simulink model "template_CR1_PreRTHS"  (Simulink 8.2)
settings: Solver=FixedStepDiscrete  StartTime=0.0  StopTime=RunningTime  FixedStep=sample  RelTol=1e-3
undefined symbols (not defined in the file): ElementsStruct, Integrator, NumFreeDOF, RigidLinkMasterMatrix, RigidLinkNo, RigidLinkNodeID, RigidLinkSlaveMatrix, sample, SampleRate, Structure
libraries: HybridFEMLibrary x2
(part 2 of 2)

== matlab function Numerical Element Calculations ==
  data: Total_RF output double; NumFreeDOF parameter double; Displacement input double; Velocity input double; ElementsStruct parameter Bus: ElementStructBus; RigidLinkNo parameter double; RigidLinkNodeID parameter double; RigidLinkMasterMatrix parameter double; RigidLinkSlaveMatrix parameter double; ElementRFs output Bus: ElementRecorderBus
% Get restoring force for each element
% Returns (6x1) restoring force vector of all elements in global coordinates %*fs
function [Total_RF,ElementRFs] = eml(NumFreeDOF, Displacement, Velocity, ElementsStruct, RigidLinkNo, RigidLinkNodeID, RigidLinkMasterMatrix, RigidLinkSlaveMatrix) %*fe
    % Store the Elements in memory
    persistent Elements;
    persistent TotalRF;        
    if isempty(Elements)
        Elements = ElementsStruct;        
    end
    
    % Storage for the Global Restoring Force        
    TotalRF = zeros(NumFreeDOF, 1);     
    ElementRFs = struct;   
    ElementRFs.Recorders = 0;
    
%Elements  %*s
[Elements.Element1, ElementRF] = GetRestoringForce_Type6(Elements.Element1, Displacement, RigidLinkNo, RigidLinkNodeID, RigidLinkMasterMatrix, RigidLinkSlaveMatrix);
TotalRF = AssembleElementGlobalRF6DOF(Elements.Element1, ElementRF, TotalRF);
[Elements.Element2, ElementRF] = GetRestoringForce_Type6(Elements.Element2, Displacement, RigidLinkNo, RigidLinkNodeID, RigidLinkMasterMatrix, RigidLinkSlaveMatrix);
TotalRF = AssembleElementGlobalRF6DOF(Elements.Element2, ElementRF, TotalRF);
[Elements.Element3, ElementRF] = GetRestoringForce_Type6(Elements.Element3, Displacement, RigidLinkNo, RigidLinkNodeID, RigidLinkMasterMatrix, RigidLinkSlaveMatrix);
TotalRF = AssembleElementGlobalRF6DOF(Elements.Element3, ElementRF, TotalRF);
[Elements.Element4, ElementRF] = GetRestoringForce_Type6(Elements.Element4, Displacement, RigidLinkNo, RigidLinkNodeID, RigidLinkMasterMatrix, RigidLinkSlaveMatrix);
TotalRF = AssembleElementGlobalRF6DOF(Elements.Element4, ElementRF, TotalRF);
[Elements.Element5, ElementRF] = GetRestoringForce_Type4(Elements.Element5, Displacement, RigidLinkNo, RigidLinkNodeID, RigidLinkMasterMatrix, RigidLinkSlaveMatrix);
TotalRF = AssembleElementGlobalRF6DOF(Elements.Element5, ElementRF, TotalRF);

%*e
                         
    Total_RF = TotalRF;


end


%%%%%%%%%%%%%%%%%%%%%%%%%%%%%%%%%%%%%%%%%%%%%%%%%%%%%%%%%%%%%%%%%%%%%%%%%%%
function TotalRF = AssembleElementGlobalRF6DOF(Element, ElementRF, TotalRF)
    % Assemble the structure restoring force vector based on the
    % degrees of freedom node locations.  
    ndof = 6;
    dof6 = zeros(6,1); 
    dof6(1,1)=Element.Nodes(1).UX;
    dof6(2,1)=Element.Nodes(1).UY;
    dof6(3,1)=Element.Nodes(1).THETA;
    dof6(4,1)=Element.Nodes(2).UX;
    dof6(5,1)=Element.Nodes(2).UY;
    dof6(6,1)=Element.Nodes(2).THETA;      

    % Add to the TotalRF    
    i = 1;
    for i=1:ndof
        if dof6(i,1) ~= -1
          TotalRF(dof6(i,1), 1) = ElementRF(i, 1) + TotalRF(dof6(i,1), 1);
        end
    end    
end

function TotalRF = AssembleElementGlobalRF9DOF(Element, ElementRF, TotalRF)
    % Assemble the structure restoring force vector based on the
    % degrees of freedom node locations.  
    ndof = 12;
    dof12 = zeros(12,1); 
    dof12(1,1)=Element.Nodes(1).UX;
    dof12(2,1)=Element.Nodes(1).UY;
    dof12(3,1)=Element.Nodes(1).THETA;
    dof12(4,1)=Element.Nodes(2).UX;
    dof12(5,1)=Element.Nodes(2).UY;
    dof12(6,1)=Element.Nodes(2).THETA;  
    dof12(7,1)=Element.Nodes(3).UX;
    dof12(8,1)=Element.Nodes(3).UY;
    dof12(9,1)=Element.Nodes(3).THETA;
    dof12(10,1)=Element.Nodes(4).UX;
    dof12(11,1)=Element.Nodes(4).UY;
    dof12(12,1)=Element.Nodes(4).THETA;

    % Add to the TotalRF
    for i=1:ndof
        if dof12(i,1) ~= -1
          TotalRF(dof12(i,1), 1) = ElementRF(i, 1) + TotalRF(dof12(i,1), 1);
        end
    end    
end

%% Element 1
function [Element, RestoringForce] = GetRestoringForce_Type1(Element, Displacement, RigidLinkNo, RigidLinkNodeID, RigidLinkMasterMatrix, RigidLinkSlaveMatrix)
    % Get distance between nodes
    X21 = Element.Nodes(2).Xcoord - Element.Nodes(1).Xcoord;
    Y21 = Element.Nodes(2).Ycoord - Element.Nodes(1).Ycoord;
    EL = sqrt(X21 * X21 + Y21 * Y21);
    EAL = Element.Material.E * Element.Area / EL;
    EIZL = Element.Material.E * Element.Inertia / EL;    
    % Calculation of density (the uniform load is only taken into account)
    SEP = zeros(6);
    SEP(1, 1) = EAL;
    SEP(1, 4) = -EAL;
    SEP(4, 4) = EAL;
    SEP(2, 2) = 12 * EIZL / EL ^ 2;
    SEP(2, 3) = 6 * EIZL / EL;
    SEP(2, 5) = -SEP(2, 2);
    SEP(2, 6) = SEP(2, 3);
    SEP(3, 3) = 4 * EIZL;
    SEP(3, 5) = -6 * EIZL / EL;
    SEP(3, 6) = 2 * EIZL;
    SEP(5, 5) = 12 * EIZL / EL ^ 2;
    SEP(5, 6) = -6 * EIZL / EL;
    SEP(6, 6) = 4 * EIZL;
    for i = 1:6
       for j = i:6
          SEP(j, i) = SEP(i, j);
       end
    end
    DCOS = zeros(3);
    DCOS(1, 1) = X21 / EL;
    DCOS(1, 2) = Y21 / EL;
    DCOS(1, 3) = 0;
    DCOS(2, 1) = -DCOS(1, 2);
    DCOS(2, 2) = DCOS(1, 1);
    DCOS(2, 3) = 0;
    DCOS(3, 1) = 0;
    DCOS(3, 2) = 0;
    DCOS(3, 3) = 1;
    ALMBDA = zeros(6);       
    for i = 1:2
       IK = 3 * (i - 1);
       for j = 1:3
          for k = 1:3
             ALMBDA(j + IK, k + IK) = DCOS(j, k);
          end
       end
    end
    SE = ALMBDA' * SEP * ALMBDA;
    % Create the displacement Ue (6x1) vector of the element in global coordinates
    Ue = zeros(6,1);
    dof = zeros(6,1);
    dof(1,1)=Element.Nodes(1).UX;
    dof(2,1)=Element.Nodes(1).UY;
    dof(3,1)=Element.Nodes(1).THETA;
    dof(4,1)=Element.Nodes(2).UX;
    dof(5,1)=Element.Nodes(2).UY;
    dof(6,1)=Element.Nodes(2).THETA;
    
    for i=1:6
        if dof(i,1) ~= -1
            Ue(i,1)=Displacement(dof(i,1),1);
        end
    end

    % Calculation Restoring Force, considering the Rigid Links if used
    if( RigidLinkNo )
        TR = RigidLinkTransformation2Nodes(Element.Nodes(1).ID, Element.Nodes(2).ID, RigidLinkNo, RigidLinkNodeID, RigidLinkMasterMatrix, RigidLinkSlaveMatrix);
        RestoringForce = TR' * SE * TR * Ue;  % (6x1) resisting force vector of element in global coordinates
    else        
        RestoringForce = SE * Ue;  % (6x1) resisting force vector of element in global coordinates
    end
end

%% Element 2
function [Element, RestoringForce] = GetRestoringForce_Type2(Element, Displacement, RigidLinkNo, RigidLinkNodeID, RigidLinkMasterMatrix, RigidLinkSlaveMatrix)
    % Preset arrays
    SE = zeros(6,6);
    SE(1, 1) = Element.Stiffness;
    SE(1, 4) = -Element.Stiffness;
    SE(4, 4) = Element.Stiffness;
    SE(4, 1) = SE(1,4);
    
    % Create the displacement Ue (6x1) vector of the element in global coordinates
    Ue = zeros(6,1);
    dof = zeros(6,1);
    dof(1,1)=Element.Nodes(1).UX;
    dof(2,1)=Element.Nodes(1).UY;
    dof(3,1)=Element.Nodes(1).THETA;
    dof(4,1)=Element.Nodes(2).UX;
    dof(5,1)=Element.Nodes(2).UY;
    dof(6,1)=Element.Nodes(2).THETA;
    
    for i=1:6
        if dof(i,1) ~= -1
            Ue(i,1)=Displacement(dof(i,1),1);
        end
    end

    % Calculation Restoring Force, considering the Rigid Links if used
    if( RigidLinkNo )
        TR = RigidLinkTransformation2Nodes(Element.Nodes(1).ID, Element.Nodes(2).ID, RigidLinkNo, RigidLinkNodeID, RigidLinkMasterMatrix, RigidLinkSlaveMatrix);
        RestoringForce = TR' * SE * TR * Ue;  % (6x1) resisting force vector of element in global coordinates
    else
%         if (RUNMODE_BIT)
%             RestoringForce = zeros(6,1);
%             RestoringForce(1,1) = Element2Input;
%             RestoringForce(4,1) = -Element2Input;
%         else
            RestoringForce = SE * Ue;  % (6x1) resisting force vector of element in global coordinates
%         end
    end    
end

%% Element 3

%% Element 4
function [Element, RestoringForce] = GetRestoringForce_Type4(Element, Displacement, RigidLinkNo, RigidLinkNodeID, RigidLinkMasterMatrix, RigidLinkSlaveMatrix)

    % element geometry       
    % element deformation % geometry restricted to 1,2 plane (x,y)
    dx = Element.xyj(1,1) - Element.xyi(1,1); 
    dy = Element.xyj(2,1) - Element.xyi(2,1);
    L = sqrt(dx*dx+dy*dy);
    dx = dx / L;
    dy = dy / L;

    % 6x6 transformation matrix from local to global coordiante
    apq  = zeros(6);
    apq(1,1) = dx; apq(2,2) = dx; apq(4,4) = dx; apq(5,5)= dx;
    apq(1,2) = dy; apq(2,1) =-dy; apq(4,5) = dy; apq(5,4)=-dy;
    apq(3,3) = 1.0; apq(6,6) =1.0;

    % element stiffness matrix in local coordinate
    SE = zeros(6,6);  
    SE(2, 2) = Element.K22;
    SE(2, 5) = Element.K25;
    SE(5, 2) = Element.K52;
    SE(5, 5) = Element.K55;
    % transformed element stiffness matrix in global coordinate
    SE = apq' * SE * apq;

    % Create the displacement Ue (6x1) vector of the element in global coordinates
    Ue = zeros(6,1);
    dof = zeros(6,1);
    dof(1,1)=Element.Nodes(1).UX;
    dof(2,1)=Element.Nodes(1).UY;
    dof(3,1)=Element.Nodes(1).THETA;
    dof(4,1)=Element.Nodes(2).UX;
    dof(5,1)=Element.Nodes(2).UY;
    dof(6,1)=Element.Nodes(2).THETA;

    for i=1:6
        if dof(i,1) ~= -1
            Ue(i,1) = Displacement(dof(i,1),1);
        end
    end
    
    % Calculation Restoring Force, considering the Rigid Links if used
    if( RigidLinkNo )
        TR = RigidLinkTransformation2Nodes(Element.Nodes(1).ID, Element.Nodes(2).ID, RigidLinkNo, RigidLinkNodeID, RigidLinkMasterMatrix, RigidLinkSlaveMatrix);
        RestoringForce = TR' * SE * TR * Ue;  % (6x1) resisting force vector of element in global coordinates
    else
        RestoringForce = SE * Ue;  % (6x1) resisting force vector of element in global coordinates
    end
end

%% Element 5

%% Element 6
function [Element,RestoringForce] = GetRestoringForce_Type6(Element, Displacement, RigidLinkNo, RigidLinkNodeID, RigidLinkMasterMatrix, RigidLinkSlaveMatrix)
    % Get the displacement Ue (6x1) vector of the element in global coordinates
    Ue = zeros(6,1);
    dof=zeros(6,1);
    dof(1,1)=Element.Nodes(1).UX;
    dof(2,1)=Element.Nodes(1).UY;
    dof(3,1)=Element.Nodes(1).THETA;
    dof(4,1)=Element.Nodes(2).UX;
    dof(5,1)=Element.Nodes(2).UY;
    dof(6,1)=Element.Nodes(2).THETA;
    for i=1:6
        if dof(i,1) ~= -1
            Ue(i,1)=Displacement(dof(i,1),1);
        end
    end

    % Calculation Restoring Force, considering the Rigid Links if used
    if( RigidLinkNo )
        TR = RigidLinkTransformation2Nodes(Element.Nodes(1).ID, Element.Nodes(2).ID, RigidLinkNo, RigidLinkNodeID, RigidLinkMasterMatrix, RigidLinkSlaveMatrix);        
        Ue = TR * Ue; 
    end       

    du=Ue-Element.Uprev;  % The incremental displacement vector du of the element in global coordinates 
    Element.Uprev=Ue; %Update Uprev of element for use in next state determination call

    % Incremental basic deformations
    dv = Element.avq * du;      

    % Integrate basic force and basic stiffness matrix
    kb = zeros(3);
    s  = zeros(3,1);

    for i=1:length(Element.sections)

        % Form B matrix and compute section deformation
        B = [ Element.b1(i) Element.b2(i) 0; 0 0 Element.b3(i) ];
        dvs = B * dv;  

        % Section state determination and update section state
        [ss ks Element.sections(i)] = SectionState( Element.sections(i), dvs );

        % Sum section term
        kb = kb + B'*ks*B * ( Element.wi(i) * Element.L/2 );
        s  = s  + B'*ss   * ( Element.wi(i) * Element.L/2 );

    end

    % Restoring force and stiffness matrix
    RestoringForce = Element.avq' * s;

    if( RigidLinkNo )
        RestoringForce = TR' * RestoringForce;  
    end
end

%% Element 7
function [Element,RestoringForce] = GetRestoringForce_Type7(Element, Displacement, RigidLinkNo, RigidLinkNodeID, RigidLinkMasterMatrix, RigidLinkSlaveMatrix, maxIter, EAT, ERT, CO)
    % Get the displacement Ue (6x1) vector of the element in global coordinates
    Ue = zeros(6,1);
    dof=zeros(6,1);
    dof(1,1)=Element.Nodes(1).UX;
    dof(2,1)=Element.Nodes(1).UY;
    dof(3,1)=Element.Nodes(1).THETA;
    dof(4,1)=Element.Nodes(2).UX;
    dof(5,1)=Element.Nodes(2).UY;
    dof(6,1)=Element.Nodes(2).THETA;
    for i=1:6
        if dof(i,1) ~= -1
            Ue(i,1)=Displacement(dof(i,1),1);
        end
    end

    % Calculation Restoring Force, considering the Rigid Links if used
    if( RigidLinkNo )
        TR = RigidLinkTransformation2Nodes(Element.Nodes(1).ID, Element.Nodes(2).ID, RigidLinkNo, RigidLinkNodeID, RigidLinkMasterMatrix, RigidLinkSlaveMatrix);        
        Ue = TR * Ue; 
    end       

    du=Ue -Element.Uprev; % The incremental displacement vector du of the element in global coordinates 


    Element.Uprev=Ue; %Update Uprev of element for use in next state determination call

    % element defomration % geometry restricted to 1,2 plane (x,y)
    dx = Element.xyj(1,1) - Element.xyi(1,1); 
    dy = Element.xyj(2,1) - Element.xyi(2,1);
    L = sqrt(dx*dx+dy*dy);
    dx = dx / L;
    dy = dy / L;

    % Form transformation matrix from element in global coordinate to basic system
    avq  = [ -dy/L  dx/L  1.  dy/L -dx/L  0;
           -dy/L  dx/L  0  dy/L -dx/L  1.;
           -dx   -dy    0  dx    dy    0];

    % Incremental basic deformations
    dv = avq * du;

    % Basic forces from previous load step
    si = Element.si; %momentI, momentJ, axial

    % Initialize ds for iteration
    ds = zeros(3,1); %deltaMomentI, deltaMomentJ, deltaAxial

    % Interpolation functions for equilibrium evaluated at integration points
    x  = (  Element.xi + 1. ) / 2.;   
    b1 = -( 1. - x );
    b2 =        x;      
    b3 = -1./L;
    b4 = ones(size(x));

    % initialize incremental section deformations
    dvsecs = zeros(2,Element.nIP);

    %vr = dv;

    % Iterate to satisfy compatibility 
    for k =1:Element.maxIter

        % Compute residual and basic flexibility by summing 
        % section properties over element length
        vr = dv;
        fb = zeros(3);
        si = Element.si; %momentI, momentJ, axial
        % loop over each section along the element length
        for i=1:Element.nIP

            % transformaion matrix 
            b = [ b1(i) b2(i) 0;
                   0     0    b4(i)];
           %        b3    b3    0]; 
            % section force, moment, axial, and shear 
            ss = b * ( ds + si );

            %%%%%%%%%%%%%%%%%%%%%%%%%%%%%%%%%%%%%%%%%%%%%%%%%%%%
            % Given section force, determine section deformation iteratively
            % Initialize vector of dvs for iteration   
             dvs = zeros(2,1);

            % Iterate on section equilibrium
      %      for j=1:Element.maxIter

                % given section deformation, determine section force
                [jthss, ks] = SectionState(Element.sections(i), dvs);            
                % residual section force 
                sres     = ss - jthss;
                dvs = ks \ sres + dvs;    



      %      end
            %%%%%%%%%%%%%%%%%%%%%%%%%%%%%%%%%%%%%%%%%%%%%%%%%%%
            % store deformation of each section
            dvsecs(:,i) = dvs;				
            % add section contribution to residual element deformation and flexibility
            vr = vr - b' * dvs   * ( Element.wi(i) * L/2. );
            fb = fb + b'*(ks\b) * ( Element.wi(i) * L/2. ); 


        end

        % check residual deformation 
    %     TolFinal=min(Element.EAT,Element.ERT1*norm(vr));
    %     if norm(vr) < TolFinal
    %         Element.NumIter=k;
    %         Element.EC=Element.EC+1;
    % 		break;
    %     end

    % check Unbalanced force   
      UnbForce=fb\vr;
      NormUnb=((UnbForce(1)*L)^2+(UnbForce(2)*L)^2+(UnbForce(3))^2)^0.5;
      TolFinal=max(Element.EAT,Element.ERT1*NormUnb);
        if NormUnb < TolFinal
            Element.NumIter=k;
            Element.EC=Element.EC+1;
            Element.NUnbforce=NormUnb;
            break;
        end
    if Element.CO==1
        ds = fb \ vr + ds; 
    end
     Element.NumIter=Element.maxIter;  
    end

    % update section state with converged dvs
    for i=1:Element.nIP
        [ssc, ksc, Element.sections(i)] = SectionState(Element.sections(i),...
            dvsecs(:,i));    
    end

    % update basic forces for element
    Element.si = ds + si;

    % Restoring force and stiffness matrix
RestoringForce = avq' * Element.si;
            
    if( RigidLinkNo )
        RestoringForce = TR' * RestoringForce;  
    end    
end


%% Element 8
function [Element,RestoringForce] = GetRestoringForce_Type8(Element, Displacement, Velocity, RigidLinkNo, RigidLinkNodeID, RigidLinkMasterMatrix, RigidLinkSlaveMatrix)
    % Get the displacement Ue (6x1) vector of the element in global coordinates
    Uev = zeros(6,1);
    Vev = zeros(6,1);
    dof=zeros(6,1);
    dof(1,1)=Element.Nodes(1).UX;
    dof(2,1)=Element.Nodes(1).UY;
    dof(3,1)=Element.Nodes(1).THETA;
    dof(4,1)=Element.Nodes(2).UX;
    dof(5,1)=Element.Nodes(2).UY;
    dof(6,1)=Element.Nodes(2).THETA;
    for i=1:6
        if dof(i,1) ~= -1
            Uev(i,1)=Displacement(dof(i,1),1);
            Vev(i,1)=Velocity(dof(i,1),1);        
        end
    end

    % Calculation Restoring Force, considering the Rigid Links if used
    if( RigidLinkNo )
        TR = RigidLinkTransformation2Nodes(Element.Nodes(1).ID, Element.Nodes(2).ID, RigidLinkNo, RigidLinkNodeID, RigidLinkMasterMatrix, RigidLinkSlaveMatrix);        
        Uev = TR * Uev; 
        Vev = TR * Vev; 
    end 

    % Deformation and velocity
    % if Element.dof ==1
    Ue = Uev(Element.dof,1)-Uev(Element.dof+3,1);
    Ve = Vev(Element.dof,1)-Vev(Element.dof+3,1);
    % elseif Element.dof ==2
    %     Ue = Uev(2,1)-Uev(5,1);
    %     Ve = Vev(2,1)-Vev(5,1);
    % else
    %     Ue = Uev(3,1)-Uev(6,1);
    %     Ve = Vev(3,1)-Vev(6,1);
    % end

    % Incremental displacement and velocity
    % the incremental deformation of the element 
    % Update max and min deformation history
    % Element.prop.Dmax= max(Ue,Element.prop.Dmax); 
    % Element.prop.Dmin= min(Ue,Element.prop.Dmin); 
    du = Ue - Element.Uprev;
    [Element.prop kt Fs] = MaterialState(du, Element.prop, Ve);

    RestoringForce=zeros(6,1);
    RestoringForce(Element.dof,1)   = Fs;
    RestoringForce(Element.dof+3,1) = -Fs;

    if( RigidLinkNo )
        RestoringForce = TR' * RestoringForce;  
    end

    % Update Uprev
    Element.Uprev=Ue; 
end


%% Element 9
function [Element,RestoringForce] = GetRestoringForce_Type9(Element, Displacement, RigidLinkNo, RigidLinkNodeID, RigidLinkMasterMatrix, RigidLinkSlaveMatrix)

%% Get the displacement Ue (12x1) vector of the element in global coordinates
ndof=12;  
Ue = zeros(ndof,1);
dof=zeros(ndof,1);
dof(1,1)=Element.Nodes(1).UX;
dof(2,1)=Element.Nodes(1).UY;
dof(3,1)=Element.Nodes(1).THETA;
dof(4,1)=Element.Nodes(2).UX;
dof(5,1)=Element.Nodes(2).UY;
dof(6,1)=Element.Nodes(2).THETA;
dof(7,1)=Element.Nodes(3).UX;
dof(8,1)=Element.Nodes(3).UY;
dof(9,1)=Element.Nodes(3).THETA;
dof(10,1)=Element.Nodes(4).UX;
dof(11,1)=Element.Nodes(4).UY;
dof(12,1)=Element.Nodes(4).THETA;

for i=1:ndof
    if dof(i,1) ~= -1
        Ue(i,1)=Displacement(dof(i,1),1);
    end
end

% Calculation Restoring Force, considering the Rigid Links if used
if( RigidLinkNo )
    TR = RigidLinkTransformation4Nodes(Element.Nodes(1).ID, Element.Nodes(2).ID, Element.Nodes(3).ID, Element.Nodes(4).ID, RigidLinkNo, RigidLinkNodeID, RigidLinkMasterMatrix, RigidLinkSlaveMatrix);        
    Ue = TR * Ue; 
end   

% The incremental displacement vector du of the element in global coordinates
% The element has 12 dofs
% Update Uprev of element for use in next state determination call
du=Ue-Element.Uprev;  
Element.Uprev=Ue; 

% transform global node displacement to basic deformation
v = Element.avq*Ue;

% compute element force
s = zeros(9,1); 

s(1) = Element.kb1*v(1);
s(2) = Element.kb2*v(2);
s(4) = Element.kb4*v(4);
s(5) = Element.kb5*v(5);
s(6) = Element.kb6*v(6);
s(7) = Element.kb7*v(7);
s(8) = Element.kb8*v(8);
s(9) = Element.kb9*v(9);

dv3 = Element.dx/Element.Width*du(10)-Element.dy/Element.Width*du(5)-Element.dx/Element.Width*du(4)+Element.dy/Element.Width*du(11)-Element.Height/Element.Width*Element.dx/Element.Width*du(2)...
    +Element.Height/Element.Width*Element.dy/Element.Width*du(1)+Element.Height/Element.Width*Element.dx/Element.Width*du(8)-Element.Height/Element.Width*Element.dy/Element.Width*du(7);

% compute shear deformation mode
[Element.ShearProp , tmp, s(3)]= MaterialState(dv3, Element.ShearProp, 0);

% Restoring force and stiffness matrix
RestoringForce = Element.avq' * s;

if( RigidLinkNo )
    RestoringForce = TR' * RestoringForce;  
end

% function [pro] = trilinear(dx, pro)
% 
% % calculate current deformation 
%     x = pro.xprev + dx; 
% 
% if pro.YieldCode == 0
% 
% 	pro.Fs1 = pro.Fs1+pro.K1*dx;
%     pro.Fs2 = pro.Fs2+pro.K2*dx;
% 	% if it is beyond elastic range, limit to yield force
% 	% and set m_nYieldCode to 1
% 	if pro.Fs1 > pro.Fy1
% 		
%         pro.Fs1 = pro.Fy1 ;
% 		pro.YieldCode = 1;
%         
%         if(pro.Fs2> pro.Fy2)
% 			pro.Fs2 = pro.Fy2 ;
% 		    pro.YieldCode = 2;
%         end
%     elseif pro.Fs1 < -pro.Fy1
% 		
%         pro.Fs1 = -pro.Fy1;
% 		pro.YieldCode = 1 ;
%        
% 		if pro.Fs2 < -pro.Fy2
% 			pro.Fs2 = - pro.Fy2 ;
% 		    pro.YieldCode = 2;
%         end
%     end
% % 1st post-yielding region    
% elseif pro.YieldCode == 1
%     
%     % assume spring2 remain elastic
%     pro.Fs2= pro.Fs2+pro.K2*dx;
%     
%     % keep loading
%     if pro.Fs1*dx > 0.
%         if pro.Fs2 > pro.Fy2
%             pro.Fs2 = pro.Fy2;
%             pro.YieldCode=2;            
%         elseif pro.Fs2 < -pro.Fy2
%             pro.Fs2 = -pro.Fy2;
%             pro.YieldCode=2;
%         end
%         % unloading
%     elseif pro.Fs1*dx < 0.
%         pro.Fs1= pro.Fs1 + pro.K1*dx;
%         pro.YieldCode = 0;
%         
%         if pro.Fs1 < -pro.Fy1 
%             pro.Fs1 = -pro.Fy1;
%             pro.YieldCode = 1;
%             if pro.Fs2 < -pro.Fy2
%                 pro.Fs2 = -pro.Fy2;
%                 pro.YieldCode = 2;
%             end
%         elseif pro.Fs1 > pro.Fy1
%             pro.Fs1 = pro.Fy1;
%             pro.YieldCode = 1;
%             if pro.Fs2 > pro.Fy2
%                 pro.Fs2 = pro.Fy2;
%                 pro.YieldCode = 2;
%             end
%         end
%     end
% elseif pro.YieldCode ==2
%     % unloading
% 	if (pro.Fs1*dx) < 0.
% 		pro.Fs1 = pro.Fs1 + pro.K1*dx;
% 		pro.Fs2 = pro.Fs2 + pro.K2*dx;
% 		pro.YieldCode = 0;
% 		
%         if pro.Fs1 < -pro.Fy1
%             pro.Fs1 = -pro.Fy1;
% 			pro.YieldCode = 1;
%             if pro.Fs2 < -pro.Fy2
% 				pro.Fs2 = -pro.Fy2;
% 				pro.YieldCode = 2;
%             end            
%         elseif pro.Fs1 > pro.Fy1
% 			pro.Fs1 = pro.Fy1;
% 			pro.YieldCode = 1;
%             if pro.Fs2> pro.Fy2
% 				pro.Fs2 = pro.Fy2;
% 				pro.YieldCode = 2;
% 			end
%         end
%     end
% end
% 
% pro.Fs = pro.Fs1 + pro.Fs2 + pro.K3*x;
% 
% % updata current state for next time step
% if pro.YieldCode == 0
%     pro.Kt = pro.K1 +pro.K2 +pro.K3;
% elseif pro.YieldCode == 1
%     pro.Kt = pro.K2 +pro.K3;    
% else
%     pro.Kt = pro.K3;
% end
% pro.xprev = x;

end
    

%%%%%%%%%%%%%%%%%%%%%%%%%%%%%%%%%%%%%%%%%%%%%%%%%%%%%%%%%%%%%%%%%%%%%%%%%%%
%%%%%%%%%%%%%%%%%%%%%%%%%%%% Helper Functions %%%%%%%%%%%%%%%%%%%%%%%%%%%%%
%%%%%%%%%%%%%%%%%%%%%%%%%%%%%%%%%%%%%%%%%%%%%%%%%%%%%%%%%%%%%%%%%%%%%%%%%%%

%% Rigid Link Tranformation Matrix Calculation for 2 Nodes, 6 DOF
function TR = RigidLinkTransformation2Nodes(Node1ID, Node2ID, RigidLinkNo, RigidLinkNodeID, RigidLinkMasterMatrix, RigidLinkSlaveMatrix)
    % Rigid Link Calculations
    TR = eye(6,6); % Transformation matrix for rigid link
    if( RigidLinkNo )    
        % Find the row with the slave node, if it exists in the element
        idx = 0;
        for kk = 1:RigidLinkNo
            if (RigidLinkNodeID(kk,2) == Node1ID)
                idx = kk;
                break;
            end
        end
        %idx=find(RigidLinkNodeID(:,2) == Node1ID); % find if a slave node exists in the element
        if ( idx )
            TL=CalculateRigidLinkTransformation(RigidLinkMasterMatrix(idx,2),RigidLinkMasterMatrix(idx,3),RigidLinkSlaveMatrix(idx,2),RigidLinkSlaveMatrix(idx,3));
            jjj = 1; % Node 1
            TR(3*(jjj-1)+1:3*jjj,3*(jjj-1)+1:3*jjj) = TL;
        end
        idx = 0;
        for kk = 1:RigidLinkNo
            if (RigidLinkNodeID(kk,2) == Node2ID)
                idx = kk;
                break;
            end
        end    
        %idx=find(RigidLinkNodeID(:,2) == Node2ID); % find if a slave node exists in the element
        if ( idx )
            TL=CalculateRigidLinkTransformation(RigidLinkMasterMatrix(idx,2),RigidLinkMasterMatrix(idx,3),RigidLinkSlaveMatrix(idx,2),RigidLinkSlaveMatrix(idx,3));            
            jjj = 2; % Node 2
            TR(3*(jjj-1)+1:3*jjj,3*(jjj-1)+1:3*jjj) = TL;
        end            
    end
end

%% Rigid Link Tranformation Matrix Calculation for 4 Nodes, 12 DOF
function TR = RigidLinkTransformation4Nodes(Node1ID, Node2ID, Node3ID, Node4ID, RigidLinkNo, RigidLinkNodeID, RigidLinkMasterMatrix, RigidLinkSlaveMatrix)
    % Rigid Link Calculations
    TR = eye(12,12); % Transformation matrix for rigid link
    if( RigidLinkNo )    
        % Find the row with the slave node, if it exists in the element
        idx = 0;
        for kk = 1:RigidLinkNo
            if (RigidLinkNodeID(kk,2) == Node1ID)
                idx = kk;
                break;
            end
        end
        %idx=find(RigidLinkNodeID(:,2) == Node1ID); % find if a slave node exists in the element
        if ( idx )
            TL=CalculateRigidLinkTransformation(RigidLinkMasterMatrix(idx,2),RigidLinkMasterMatrix(idx,3),RigidLinkSlaveMatrix(idx,2),RigidLinkSlaveMatrix(idx,3));
            jjj = 1; % Node 1
            TR(3*(jjj-1)+1:3*jjj,3*(jjj-1)+1:3*jjj) = TL;
        end
        idx = 0;
        for kk = 1:RigidLinkNo
            if (RigidLinkNodeID(kk,2) == Node2ID)
                idx = kk;
                break;
            end
        end    
        %idx=find(RigidLinkNodeID(:,2) == Node2ID); % find if a slave node exists in the element
        if ( idx )
            TL=CalculateRigidLinkTransformation(RigidLinkMasterMatrix(idx,2),RigidLinkMasterMatrix(idx,3),RigidLinkSlaveMatrix(idx,2),RigidLinkSlaveMatrix(idx,3));            
            jjj = 2; % Node 2
            TR(3*(jjj-1)+1:3*jjj,3*(jjj-1)+1:3*jjj) = TL;
        end                
        % Find the row with the slave node, if it exists in the element
        idx = 0;
        for kk = 1:RigidLinkNo
            if (RigidLinkNodeID(kk,2) == Node3ID)
                idx = kk;
                break;
            end
        end
        %idx=find(RigidLinkNodeID(:,2) == Node3ID); % find if a slave node exists in the element
        if ( idx )
            TL=CalculateRigidLinkTransformation(RigidLinkMasterMatrix(idx,2),RigidLinkMasterMatrix(idx,3),RigidLinkSlaveMatrix(idx,2),RigidLinkSlaveMatrix(idx,3));
            jjj = 3; % Node 3
            TR(3*(jjj-1)+1:3*jjj,3*(jjj-1)+1:3*jjj) = TL;
        end
        idx = 0;
        for kk = 1:RigidLinkNo
            if (RigidLinkNodeID(kk,2) == Node4ID)
                idx = kk;
                break;
            end
        end    
        %idx=find(RigidLinkNodeID(:,2) == Node4ID); % find if a slave node exists in the element
        if ( idx )
            TL=CalculateRigidLinkTransformation(RigidLinkMasterMatrix(idx,2),RigidLinkMasterMatrix(idx,3),RigidLinkSlaveMatrix(idx,2),RigidLinkSlaveMatrix(idx,3));            
            jjj = 4; % Node 4
            TR(3*(jjj-1)+1:3*jjj,3*(jjj-1)+1:3*jjj) = TL;
        end          
    end
end

%% Calculate Rigid Link Transformation
function TL = CalculateRigidLinkTransformation(MNXcoord, MNYcoord, SNXcoord, SNYcoord)
    X1 = MNXcoord; Y1 = MNYcoord;
    X2 = SNXcoord;  Y2 = SNYcoord;
    deltaX = X2 - X1;
    deltaY = Y2 - Y1;
    TL = [ 1 0 -deltaY;
           0 1  deltaX;
           0 0  1    ];
end

%% State determination for fiber section
function [ss, ks, sec] = SectionState( sec, dvs )
% For section sec undergoing a change
% in section deformation dvs=[curvature strain], compute
% section forces SS=[moment axial] and the 2x2 tangents
% section stiffness KS.
    ks = zeros(2,2);
    ss = zeros(2,1);  
    numfib = length(sec.fibers);

    % Loop over fibers
    for i=1:numfib
        yi   = sec.fibers(i).yi;
        area = sec.fibers(i).A;

        % Change in strain
        deps = yi * dvs(1:2);

        [sec.fibers(i).prop Et sc] = MaterialState(deps, sec.fibers(i).prop, 0 );        

        % Integration -- add contribution of fiber 
        % for 3D --- following codes need to be modified
        ks = ks + yi'*yi * (area*Et ); % may not need to do it
        ss = ss + yi'    * (area*sc);
    end
end

%% Material Section State
function [ mat Et sc] = MaterialState( dep, mat, vc)  
    %MATERIALSTATE Summary of this function goes here
    %   dep = incremental deformation at the current time step, except for
    %   Bouc-Wen model
    %   mat = material data structure
    %   vc  = 0 for other materials
    %       = current velocity for Bouc-Wen material
    %
    switch  mat.Type
        case 2
            mat = bilinearMat(dep, mat);
            Et = mat.Et;
            sc = mat.sc;
%       case 3
        case 4
            mat = BoucWen(dep, mat, vc);
            Et = mat.k;
            sc = mat.Qj;
        case 5
            mat = trilinear(dep, mat);
            Et = mat.Kt;
            sc = mat.Fs;
%         case 6     
        case 7
            mat = Concrete01(dep, mat);
            Et = mat.Ttangent;
            sc = mat.Cstress;
        case 9
            mat = Steel02(dep, mat);
            Et = mat.e;
            sc = mat.sig;
        otherwise
            Et = 0;
            sc = 0;
    end
end

%% Bilinear Material Section State
function [mat] = bilinearMat(deps, mat )
    %	[mat]=BILINEARMAT(deps,mat) For strain increment deps
    %	and mat compute new properties for bilinear material.
    %	mat.SY, mat.E, mat.EP are the yield stress,
    %	first slop and second slope respectively.  materialProp.SC,
    %	mat.SB, materialSE are the current stress, back stress, and
    %	current strain, respectively. mat.ET is the current tangent modulus.

    % Material properties
    sigy = mat.sy;		% yield stress
    E    = mat.e;		% E
    Ep   = mat.ep;		% alpha*E

    % State from last converged load step
    sig  = mat.sc;		% stress
    sigb = mat.sb;		% backstress
    code = mat.cd;		% yield code
                        %	=0, elastic
                        %	=1, plastic

    if code==0 || ( code==1 && (sig-sigb)*deps < 0 )
        % Strain to plastic loading from elastic state
        deps1 = ( sign(deps) * sigy + sigb - sig ) / E;

        % Elastic
        sig  = sig + E * deps;
        Et   = E;
        code = 0;

        % Check if plasic loading from elastic state
        if abs(deps) > abs(deps1)
            sig  = sig  + ( Ep - E ) * ( deps - deps1 );
            sigb = sigb +   Ep       * ( deps - deps1 );
            Et   = Ep;
            code = 1;
        end

    else
        % Continue plastic loading
        sig  = sig  + Ep * deps;
        sigb = sigb + Ep * deps;
        Et   = Ep;
        code = 1;

    end

    % Return updated state. 
    mat.sc = sig;
    mat.sb = sigb;
    mat.cd = code;
    mat.es = mat.es + deps;	
    mat.Et = Et;
end   

%% BoucWen Material Section State
function [BW]= BoucWen( dx, BW, vcur)
    % ---------------------------------------------
    % x,v: displacement and velocity
    %   Q: restoring force
    %   z: hysteretic component
    %  zj: z in next step, i.e. z_i+1
    %  BW: numerous parameters for Bouc-Wen model
    %   i: step number

    xcur =  dx + BW.Uprev;
    % Fourth order R-K forward integration
    dz1 = dx*f(BW,vcur,BW.zj);
    dz2 = dx*f(BW,vcur,BW.zj+dz1/2);
    dz3 = dx*f(BW,vcur,BW.zj+dz2/2);
    dz4 = dx*f(BW,vcur,BW.zj+dz3);
    zj = BW.zj + (dz1+2*dz2+2*dz3+dz4)/6;

    umax=(abs(BW.Dmin)+ BW.Dmax)*0.5;    
    BW.k=BW.k1*exp(-umax/BW.uref) + BW.k2;    
    BW.Qj = BW.c*(abs(vcur)^BW.a)*sign(vcur) + BW.alpha*BW.k*xcur +...
        (1-BW.alpha)*BW.k*BW.uy*zj;

    % update deformation for next time step
    BW.Uprev = xcur;
    BW.Dmax= max(xcur,BW.Dmax); 
    BW.Dmin= min(xcur,BW.Dmin); 
    BW.zj =  zj;
end

% BoucWen Helper
function y=f(BW,v,z)
    % This function describes the nonlinear differential equation that governs
    % the hysteretic component, z.
    % The returned value is "dz/dx" or "z_dot/x_dot"
    y =(1/BW.uy)*(1-BW.beta*sign(v)*abs(z)^BW.n*sign(z)-BW.gamma1*abs(z)^BW.n);
end
%%%%%%%%%%%%%%%%%%% End of Bouc-Wen Model %%%%%%%%%%%%%%%%%%%%%%%% 

%% Trilinear Material Section State
function [pro] = trilinear(dx, pro)
    % calculate current deformation 
        x = pro.xprev + dx; 

    if pro.YieldCode == 0

        pro.Fs1 = pro.Fs1+pro.K1*dx;
        pro.Fs2 = pro.Fs2+pro.K2*dx;
        % if it is beyond elastic range, limit to yield force
        % and set m_nYieldCode to 1
        if pro.Fs1 > pro.Fy1

            pro.Fs1 = pro.Fy1 ;
            pro.YieldCode = 1;

            if(pro.Fs2> pro.Fy2)
                pro.Fs2 = pro.Fy2 ;
                pro.YieldCode = 2;
            end
        elseif pro.Fs1 < -pro.Fy1

            pro.Fs1 = -pro.Fy1;
            pro.YieldCode = 1 ;

            if pro.Fs2 < -pro.Fy2
                pro.Fs2 = - pro.Fy2 ;
                pro.YieldCode = 2;
            end
        end
    % 1st post-yielding region    
    elseif pro.YieldCode == 1

        % assume spring2 remain elastic
        pro.Fs2= pro.Fs2+pro.K2*dx;

        % keep loading
        if pro.Fs1*dx > 0.
            if pro.Fs2 > pro.Fy2
                pro.Fs2 = pro.Fy2;
                pro.YieldCode=2;            
            elseif pro.Fs2 < -pro.Fy2
                pro.Fs2 = -pro.Fy2;
                pro.YieldCode=2;
            end
            % unloading
        elseif pro.Fs1*dx < 0.
            pro.Fs1= pro.Fs1 + pro.K1*dx;
            pro.YieldCode = 0;

            if pro.Fs1 < -pro.Fy1 
                pro.Fs1 = -pro.Fy1;
                pro.YieldCode = 1;
                if pro.Fs2 < -pro.Fy2
                    pro.Fs2 = -pro.Fy2;
                    pro.YieldCode = 2;
                end
            elseif pro.Fs1 > pro.Fy1
                pro.Fs1 = pro.Fy1;
                pro.YieldCode = 1;
                if pro.Fs2 > pro.Fy2
                    pro.Fs2 = pro.Fy2;
                    pro.YieldCode = 2;
                end
            end
        end
    elseif pro.YieldCode ==2
        % unloading
        if (pro.Fs1*dx) < 0.
            pro.Fs1 = pro.Fs1 + pro.K1*dx;
            pro.Fs2 = pro.Fs2 + pro.K2*dx;
            pro.YieldCode = 0;

            if pro.Fs1 < -pro.Fy1
                pro.Fs1 = -pro.Fy1;
                pro.YieldCode = 1;
                if pro.Fs2 < -pro.Fy2
                    pro.Fs2 = -pro.Fy2;
                    pro.YieldCode = 2;
                end            
            elseif pro.Fs1 > pro.Fy1
                pro.Fs1 = pro.Fy1;
                pro.YieldCode = 1;
                if pro.Fs2> pro.Fy2
                    pro.Fs2 = pro.Fy2;
                    pro.YieldCode = 2;
                end
            end
        end
    end

    pro.Fs = pro.Fs1 + pro.Fs2 + pro.K3*x;

    % updata current state for next time step
    if pro.YieldCode == 0
        pro.Kt = pro.K1 +pro.K2 +pro.K3;
    elseif pro.YieldCode == 1
        pro.Kt = pro.K2 +pro.K3;    
    else
        pro.Kt = pro.K3;
    end
    pro.xprev = x;
end

%% Concrete01 Material Section State
function [mat] = Concrete01(dStrain , mat)

    % Get the total strain     
    mat.Tstrain = dStrain + mat.Cstrain;
    % Get the previous states
    mat.TminStrain = mat.CminStrain;
    mat.TendStrain = mat.CendStrain;
    mat.TunloadSlope = mat.CunloadSlope;
    mat.Tstress = mat.Cstress;
    mat.Ttangent = mat.Ctangent;        
    
    % check for a quick return
    if (mat.Tstrain > 0.0)
        mat.Tstress = 1e-10;
        mat.Ttangent = 0;%1e-10;
    end    
    
    mat.TunloadSlope = mat.CunloadSlope;  
  
    tempStress = mat.Cstress + mat.TunloadSlope*mat.Tstrain - mat.TunloadSlope*mat.Cstrain;
  
    % Material goes further into compression
    if (mat.Tstrain < mat.Cstrain)   
        mat.TminStrain = mat.CminStrain;
        mat.TendStrain = mat.CendStrain;  
    
        [mat] = reload(mat);
    
        if (tempStress > mat.Tstress) 
            mat.Tstress = tempStress;
            mat.Ttangent = mat.TunloadSlope;
        end
    
    % Material goes TOWARD tension
    elseif (tempStress <= 0.0)
        mat.Tstress = tempStress;
        mat.Ttangent = mat.TunloadSlope;
        
    % Made it into tension
    else
        mat.Tstress = 1e-10;
        mat.Ttangent = 0;%1e-10;
    end
         
    % Save states
    mat.CminStrain = mat.TminStrain;
    mat.CendStrain = mat.TendStrain;
    mat.CunloadSlope = mat.TunloadSlope;
    mat.Cstress = mat.Tstress;
    mat.Ctangent = mat.Ttangent;
    mat.Cstrain = mat.Tstrain;  
end

% Reload, Concrete01
function [mat] = reload(mat)

    if (mat.Tstrain <= mat.TminStrain)     
        mat.TminStrain = mat.Tstrain;
    
        % Determine point on envelope
        [mat] = envelope(mat);     
        [mat] = unload(mat);     
    elseif (mat.Tstrain <= mat.TendStrain) 
        mat.Ttangent = mat.TunloadSlope;
        mat.Tstress = mat.Ttangent*(mat.Tstrain-mat.TendStrain);
    else 
        mat.Tstress = 1e-10;
        mat.Ttangent = 0;%1e-10;
    end 
end
    
% Envelope, Concrete01
function [mat] = envelope(mat)  

    if (mat.Tstrain > mat.epsc0) 
        eta = mat.Tstrain/mat.epsc0;
        mat.Tstress = mat.fpc*(2*eta-eta*eta);
        Ec0 = 2.0*mat.fpc/mat.epsc0;  % changed
        mat.Ttangent = Ec0*(1.0-eta); % changed
    elseif (mat.Tstrain > mat.epscu) 
        mat.Ttangent = (mat.fpc-mat.fpcu)/(mat.epsc0-mat.epscu);
        mat.Tstress = mat.fpc + mat.Ttangent*(mat.Tstrain-mat.epsc0);
    else 
        mat.Tstress = mat.fpcu;
        mat.Ttangent = 1e-10;
    end
end

% Unload, Concrete01
function [mat] = unload(mat)   
    DBL_EPSILON=2.2204460492503131e-16;
  
    tempStrain = mat.TminStrain;
  
    if (tempStrain < mat.epscu)
        tempStrain = mat.epscu;
    end
    eta = tempStrain/mat.epsc0;
    ratio = 0.707*(eta-2.0) + 0.834;
    if (eta < 2.0)
        ratio = 0.145*eta*eta + 0.13*eta;
    end
    mat.TendStrain = ratio*mat.epsc0;
    temp1 = mat.TminStrain - mat.TendStrain;
    Ec0 = 2.0*mat.fpc/mat.epsc0;  % changed
    temp2 = mat.Tstress/Ec0;   % changed
  
    if (temp1 > -DBL_EPSILON) % temp1 should always be negative
        mat.TunloadSlope = Ec0;  % changed
    elseif (temp1 <= temp2)
        mat.TendStrain = mat.TminStrain - temp1;
        mat.TunloadSlope = mat.Tstress/temp1;
    else 
        mat.TendStrain = mat.TminStrain - temp2;
        mat.TunloadSlope = Ec0;  % changed
    end
end
%%%%%%%%%%%%%%%%%%%%%%%%End of Concrete01 Material%%%%%%%%%%%%%%%%%%%%%%%%%%%%%%%%%%%%%%%%%%%

function [mat] = Steel02(deps , mat)

  mat.Esh = mat.b*mat.E0;
  mat.epsy = mat.Fy / mat.E0;
  
  mat.eps=mat.epsP;
  mat.e = mat.eP;
  mat.sig = mat.sigP;
  mat.epsmax = mat.epsmaxP;
  mat.epsmin = mat.epsminP;
  mat.epspl  = mat.epsplP;
  mat.epss0  = mat.epss0P;  
  mat.sigs0  = mat.sigs0P; 
  mat.epsr   = mat.epssrP;  
  mat.sigr   = mat.sigsrP;  
  mat.kon = mat.konP;
  % modified C-P. Lamarche 2006
  if (mat.sigini ~= 0.0) 
    epsini = mat.sigini/mat.E0;
    mat.eps = deps + mat.epsP +epsini;
  else
  mat.eps = deps + mat.epsP;
  end
 
  
  DBL_EPSILON=2.2204460492503131e-16;
 if (mat.kon == 0 || mat.kon == 3) % modified C-P. Lamarche 2006


%     if (abs(deps) < 10.0*DBL_EPSILON)
% 
%       mat.e = mat.E0;
%       mat.sig = mat.sigini;               % modified C-P. Lamarche 2006
%       mat.kon = 3;                     % modified C-P. Lamarche 2006 flag to impose initial stess/strain
%     else 

      mat.epsmax = mat.epsy;
      mat.epsmin = -mat.epsy;
        if (deps < 0.0) 
          mat.kon = 2;
          mat.epss0 = mat.epsmin;
          mat.sigs0 = -mat.Fy;
          mat.epspl = mat.epsmin;
        else 
          mat.kon = 1;
          mat.epss0 = mat.epsmax;
          mat.sigs0 = mat.Fy;
          mat.epspl = mat.epsmax;
       end
     %end
 end
 
 if (mat.kon == 2 && deps > 0.0) 


    mat.kon = 1;
    mat.epsr = mat.epsP;
    mat.sigr = mat.sigP;
    %epsmin = min(epsP, epsmin);
    if (mat.epsP < mat.epsmin)
     mat.epsmin = mat.epsP;
    end
     d1 = (mat.epsmax - mat.epsmin) / (2.0*(mat.a4 * mat.epsy));
     shft = 1.0 + mat.a3 * (d1^0.8);
     mat.epss0 = (mat.Fy * shft - mat.Esh * mat.epsy * shft - mat.sigr + mat.E0 * mat.epsr) / (mat.E0 - mat.Esh);
     mat.sigs0 = mat.Fy * shft + mat.Esh * (mat.epss0 - mat.epsy * shft);
     mat.epspl = mat.epsmax;

 elseif (mat.kon == 1 && deps < 0.0)
    
    % update the maximum previous strain, store the last load reversal 
    % point and calculate the stress and strain (sigs0 and epss0) at the 
    % new intersection between elastic and strain hardening asymptote 
    % To include isotropic strain hardening shift the strain hardening 
    % asymptote by sigsft before calculating the intersection point 
    % Constants a1 and a2 control this stress shift on compression side 

    mat.kon = 2;
    mat.epsr = mat.epsP;
    mat.sigr = mat.sigP;
    % epsmax = max(epsP, epsmax);
    if (mat.epsP > mat.epsmax)
      mat.epsmax = mat.epsP;
    end
    d1 = (mat.epsmax - mat.epsmin) / (2.0*(mat.a2 * mat.epsy));
    shft = 1.0 + mat.a1 * (d1^0.8);
    mat.epss0 = (-mat.Fy * shft + mat.Esh * mat.epsy * shft - mat.sigr + mat.E0 * mat.epsr) / (mat.E0 - mat.Esh);
    mat.sigs0 = -mat.Fy * shft + mat.Esh * (mat.epss0 + mat.epsy * shft);
    mat.epspl = mat.epsmin;
 end
 
  xi  = abs((mat.epspl-mat.epss0)/mat.epsy);
  R   = mat.R0*(1.0 - (mat.cR1*xi)/(mat.cR2+xi));
  epsrat = (mat.eps-mat.epsr)/(mat.epss0-mat.epsr);
  dum1  = 1.0 + (abs(epsrat)^R);
  dum2  = (dum1^(1/R));

  mat.sig   = mat.b*epsrat +(1.0-mat.b)*epsrat/dum2;
  mat.sig   = mat.sig*(mat.sigs0-mat.sigr)+mat.sigr;

  mat.e = mat.b + (1.0-mat.b)/(dum1*dum2);
  mat.e = mat.e*(mat.sigs0-mat.sigr)/(mat.epss0-mat.epsr);
  
  mat.epsminP = mat.epsmin;
  mat.epsmaxP = mat.epsmax;
  mat.epsplP = mat.epspl;
  mat.epss0P = mat.epss0;
  mat.sigs0P = mat.sigs0;
  mat.epssrP = mat.epsr;
  mat.sigsrP = mat.sigr;
  mat.konP = mat.kon;
  
  mat.eP = mat.e;
  mat.sigP = mat.sig;
  mat.epsP = mat.eps;
end

== matlab function Calculate Command Vectors Type 1 CR/MATLAB Function ==
  data: Alpha1 input double; Alpha2 input double; Timestep input double; TimestepSquared input double; Acceleration input double; Displacement output double; Velocity output double; Prev_Displacement input double; Prev_Velocity input double
function [Displacement, Velocity]  = fcn(Alpha1,...
                                        Alpha2,...
                                        Timestep,...
                                        TimestepSquared,...
                                        Acceleration,...
                                        Prev_Displacement,...
                                        Prev_Velocity)
                                                
Displacement = Prev_Displacement + ...
                  Timestep * Prev_Velocity + ...
                  Alpha2 * TimestepSquared * Acceleration;

Velocity = Prev_Velocity + Alpha1 * Timestep * Acceleration;
